simulink model "bicycle_sim11"  (Simulink 8.7)
settings: Solver=VariableStepAuto  SolverMode=SingleTasking  StartTime=0.0  StopTime=30  RelTol=1e-3
values from neighbouring files (symbols this model uses):
  a = 4    [bicycle.m]    (also in diff_drive.m)
  d = 0.01    [bicycle.m]    (also in diff_drive.m = 0.075)
  K_theta = 1    [bicycle.m]    (also in diff_drive.m = 0.001)
  Kp = 7    [bicycle.m]    (also in diff_drive.m = 1)
  Kx = 30    [bicycle.m]    (also in diff_drive.m = 15)
  Ky = 30    [bicycle.m]    (also in diff_drive.m = 150)
  theta0 = pi/2    (= 1.57079632679)    [bicycle.m]    (also in diff_drive.m)
  w = 0.1    [bicycle.m]    (also in diff_drive.m)
  x0 = a    (= 4)    [bicycle.m]    (also in diff_drive.m)
  y0 = 0    [bicycle.m]    (also in diff_drive.m)
libraries: simulink_extras x2
settings Model: Creator=olivier  LastModifiedBy=sanjy
settings SolverCC: ZeroCrossAlgorithm=Adaptive
settings DataIOCC: LimitDataPoints=off  SaveFormat=Dataset
settings DebuggingCC: UnderspecifiedInitializationDetection=Simplified  MergeDetectMultiDrivingBlocksExec=error  MaskedZcDiagnostic=none  SFUnexpectedBacktrackingDiag=error  SFNoUnconditionalDefaultTransitionDiag=error
settings HardwareCC: ProdBitPerPointer=64  ProdLargestAtomicFloat=Float  ProdIntDivRoundTo=Zero  ProdEndianess=LittleEndian  ProdWordSize=64  ProdHWDeviceType=Intel->x86-64 (Windows64)
settings ModelReferenceCC: PropagateSignalLabelsOutOfModel=on
settings SFSimCC: SimUseLocalCustomCode=on
settings RTWCC: RTWUseLocalCustomCode=on
settings GRTTargetCC: TargetLangStandard=C99 (ISO)  GeneratePreprocessorConditionals=Use local settings
settings ConfigComp: CovMetricSettings=dwe  CovHtmlReporting=off  CovSaveCumulativeToWorkspaceVar=off  CovSaveSingleToWorkspaceVar=off  CovModelRefEnable=off  CovExternalEMLEnable=on

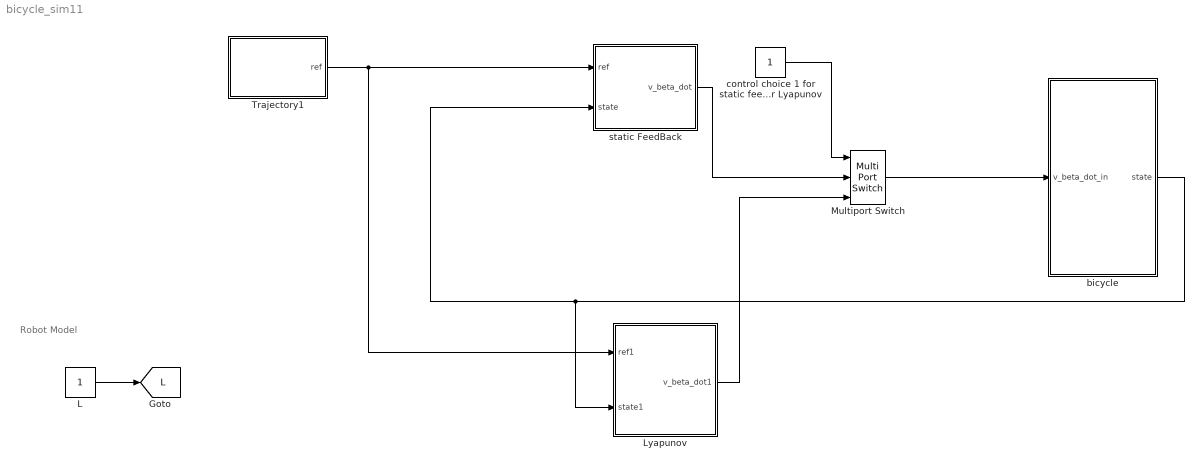
== system bicycle_sim11 ==
  note: Robot Model
  L : Constant
  Lyapunov : Subsystem
  Multiport Switch : MultiPortSwitch  Inputs=2
  Trajectory1 : Subsystem  TreatAsAtomicUnit=on
  bicycle : Subsystem  mask{L_error=0, radius_error=0, omega_max=100, beta_max=45, beta_dot_max=50}
      mask prompts: L_error "L error in percent"; radius_error "Radius error in percent"; omega_max "Max Rotation Velocity"; beta_max "Max Orientation"; beta_dot_max "Max Orientation Velocity"
  control choice 1 for static feedback 2 for Lyapunov : Constant
  static FeedBack : Subsystem
  tag scope: L=global
  wires:
  Lyapunov/1(v_beta_dot1) -> Multiport Switch/3
  L/1 -> [L]
  bicycle/1(state) -> Lyapunov/2(state1), static FeedBack/2(state)
  control choice 1 for static feedback 2 for Lyapunov/1 -> Multiport Switch/1
  Multiport Switch/1 -> bicycle/1(v_beta_dot_in)
  static FeedBack/1(v_beta_dot) -> Multiport Switch/2
  Trajectory1/1(ref) -> Lyapunov/1(ref1), static FeedBack/1(ref)

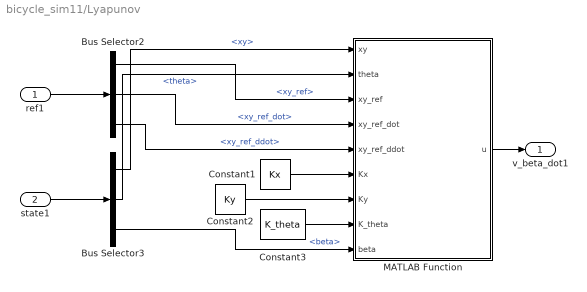
== system bicycle_sim11/Lyapunov ==
  ref1 : Inport
  state1 : Inport  Port=2
  Bus Selector2 : BusSelector  OutputSignals=xy_ref,xy_ref_dot,xy_ref_ddot
  Bus Selector3 : BusSelector  OutputSignals=xy,theta,beta
  Constant1 : Constant  Value=Kx
  Constant2 : Constant  Value=Ky
  Constant3 : Constant  Value=K_theta
  MATLAB Function : MATLAB Function  TreatAsAtomicUnit=on
  v_beta_dot1 : Outport
  wires:
  Constant3/1 -> MATLAB Function/8(K_theta)
  Constant2/1 -> MATLAB Function/7(Ky)
  Constant1/1 -> MATLAB Function/6(Kx)
  Bus Selector3/2 -> MATLAB Function/2(theta)  "<theta>"
  Bus Selector2/1 -> MATLAB Function/3(xy_ref)  "<xy_ref>"
  Bus Selector3/1 -> MATLAB Function/1(xy)  "<xy>"
  Bus Selector2/2 -> MATLAB Function/4(xy_ref_dot)  "<xy_ref_dot>"
  MATLAB Function/1(u) -> v_beta_dot1/1
  state1/1 -> Bus Selector3/1
  Bus Selector2/3 -> MATLAB Function/5(xy_ref_ddot)  "<xy_ref_ddot>"
  ref1/1 -> Bus Selector2/1
  Bus Selector3/3 -> MATLAB Function/9(beta)  "<beta>"

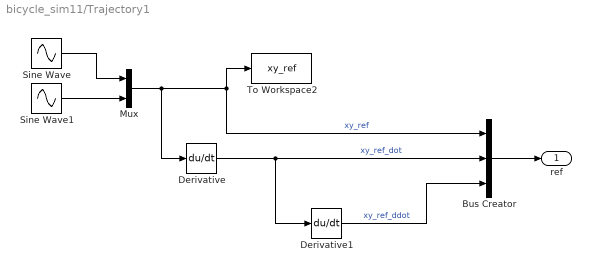
== system bicycle_sim11/Trajectory1 ==
  Bus Creator : BusCreator  Inputs=3
  Derivative : Derivative
  Derivative1 : Derivative
  Mux : Mux  Inputs=2
  Sine Wave : Sin  Amplitude=a  Frequency=w  Phase=pi/2  SampleTime=0
  Sine Wave1 : Sin  Amplitude=a  Frequency=w  SampleTime=0
  To Workspace2 : ToWorkspace  VariableName=xy_ref  SampleTime=-1
      settings: Save2DSignal=2-D array (concatenate along first dimension)
  ref : Outport
  wires:
  Bus Creator/1 -> ref/1
  Mux/1 -> Derivative/1, Bus Creator/1, To Workspace2/1  "xy_ref"
  Derivative/1 -> Bus Creator/2, Derivative1/1  "xy_ref_dot"
  Derivative1/1 -> Bus Creator/3  "xy_ref_ddot"
  Sine Wave1/1 -> Mux/2
  Sine Wave/1 -> Mux/1

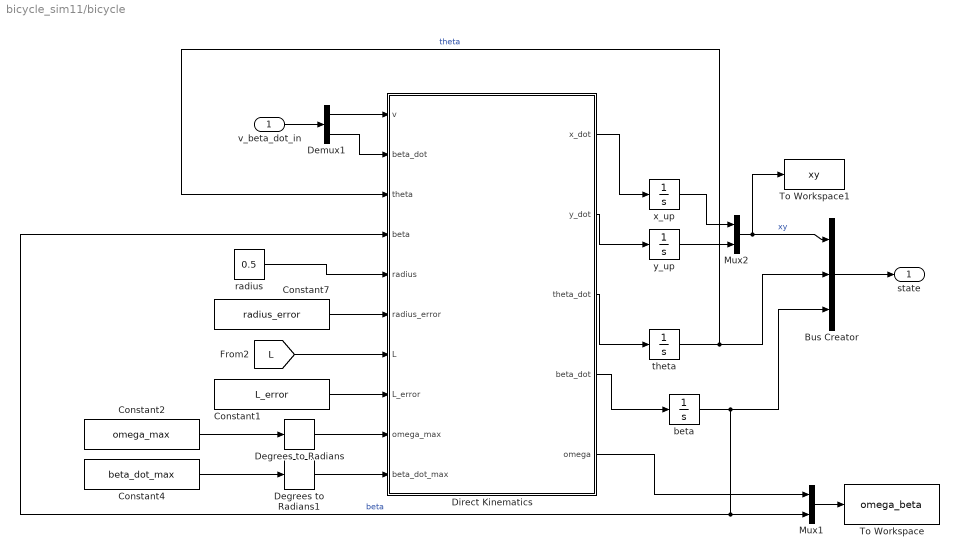
== system bicycle_sim11/bicycle ==
  v_beta_dot_in : Inport
  Bus Creator : BusCreator  Inputs=3
  Constant1 : Constant  Value=L_error
  Constant2 : Constant  Value=omega_max
  Constant4 : Constant  Value=beta_dot_max
  Constant7 : Constant  Value=radius_error
  Degrees to Radians : simulink_extras/Transformations/Degrees to Radians
  Degrees to Radians1 : simulink_extras/Transformations/Degrees to Radians
  Demux1 : Demux  Outputs=2
  Direct Kinematics : MATLAB Function  TreatAsAtomicUnit=on
  Mux1 : Mux  Inputs=2
  Mux2 : Mux  Inputs=2
  To Workspace : ToWorkspace  VariableName=omega_beta  SampleTime=-1
      settings: Save2DSignal=2-D array (concatenate along first dimension)
  To Workspace1 : ToWorkspace  VariableName=xy  SampleTime=-1
      settings: Save2DSignal=2-D array (concatenate along first dimension)
  beta : Integrator  LimitOutput=on  UpperSaturationLimit=beta_max*pi/180  LowerSaturationLimit=-beta_max*pi/180
  radius : Constant  Value=0.5
  theta : Integrator  InitialCondition=theta0
  x_up : Integrator  InitialCondition=x0
  y_up : Integrator  InitialCondition=y0
  state : Outport
  wires:
  Direct Kinematics/2(y_dot) -> y_up/1
  Direct Kinematics/1(x_dot) -> x_up/1
  x_up/1 -> Mux2/1
  y_up/1 -> Mux2/2
  Mux2/1 -> Bus Creator/1, To Workspace1/1  "xy"
  Bus Creator/1 -> state/1
  v_beta_dot_in/1 -> Demux1/1
  Demux1/1 -> Direct Kinematics/1(v)
  [L] -> Direct Kinematics/7(L)
  Constant1/1 -> Direct Kinematics/8(L_error)
  Constant7/1 -> Direct Kinematics/6(radius_error)
  Direct Kinematics/3(theta_dot) -> theta/1
  Direct Kinematics/4(beta_dot) -> beta/1
  theta/1 -> Direct Kinematics/3(theta), Bus Creator/2  "theta"
  beta/1 -> Direct Kinematics/4(beta), Mux1/2, Bus Creator/3  "beta"
  Constant2/1 -> Degrees to Radians/1
  Constant4/1 -> Degrees to Radians1/1
  Direct Kinematics/5(omega) -> Mux1/1
  Mux1/1 -> To Workspace/1
  radius/1 -> Direct Kinematics/5(radius)
  Demux1/2 -> Direct Kinematics/2("beta_dot ")
  Degrees to Radians/1 -> Direct Kinematics/9(omega_max)
  Degrees to Radians1/1 -> Direct Kinematics/10(beta_dot_max)

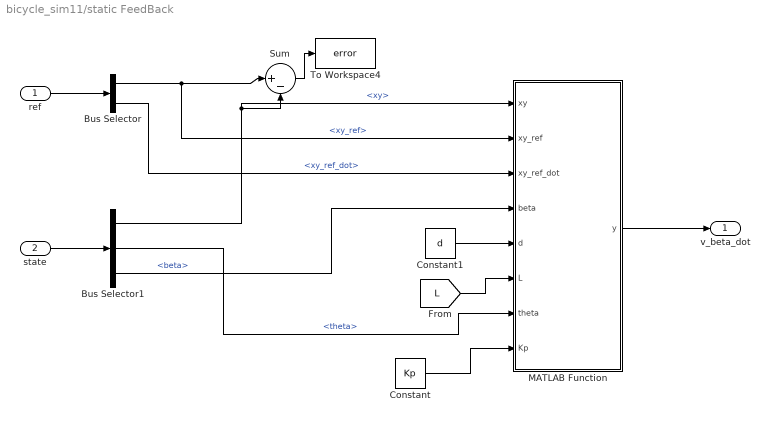
== system bicycle_sim11/static FeedBack ==
  ref : Inport
  state : Inport  Port=2
  Bus Selector : BusSelector  OutputSignals=xy_ref,xy_ref_dot
  Bus Selector1 : BusSelector  OutputSignals=xy,theta,beta
  Constant : Constant  Value=Kp
  Constant1 : Constant  Value=d
  MATLAB Function : MATLAB Function  TreatAsAtomicUnit=on
  Sum : Sum  Inputs=|+-
  To Workspace4 : ToWorkspace  VariableName=error  SampleTime=-1
      settings: Save2DSignal=2-D array (concatenate along first dimension)
  v_beta_dot : Outport
  wires:
  Sum/1 -> To Workspace4/1
  ref/1 -> Bus Selector/1
  state/1 -> Bus Selector1/1
  Bus Selector/1 -> MATLAB Function/2(xy_ref), Sum/1  "<xy_ref>"
  Bus Selector1/1 -> MATLAB Function/1(xy), Sum/2  "<xy>"
  Constant1/1 -> MATLAB Function/5(d)
  [L] -> MATLAB Function/6(L)
  Bus Selector/2 -> MATLAB Function/3(xy_ref_dot)  "<xy_ref_dot>"
  Bus Selector1/3 -> MATLAB Function/4(beta)  "<beta>"
  Bus Selector1/2 -> MATLAB Function/7(theta)  "<theta>"
  Constant/1 -> MATLAB Function/8(Kp)
  MATLAB Function/1(y) -> v_beta_dot/1

== matlab function bicycle/Direct Kinematics ==
  data: v input double; beta_dot input double; x_dot output double; theta input double; beta input double; radius input double; radius_error input double; L input double; L_error input double; omega_max input double; beta_dot_max input double; y_dot output double; theta_dot output double; beta_dot output double; omega output double
function [x_dot, y_dot, theta_dot, beta_dot, omega]  = dk(v, beta_dot, theta, beta, radius, radius_error, L, L_error, omega_max, beta_dot_max)

% commanded wheel rotation velocity
omega = v/radius;
omega = max(-omega_max, min(omega, omega_max));

% actual linear velocity
v = (1+radius_error*0.01)*radius * omega;

% actual L value
L = (1+L_error*0.01)*L;

x_dot = v*cos(theta)*cos(beta);
y_dot = v*sin(theta)*cos(beta);
theta_dot = v*sin(beta)/L;
beta_dot = max(-beta_dot_max, min(beta_dot, beta_dot_max));

== matlab function static FeedBack/MATLAB Function ==
  data: xy input double; y output double; xy_ref input double; xy_ref_dot input double; beta input double; d input double; L input double; theta input double; Kp input double
function y = fcn(xy,xy_ref,xy_ref_dot,beta,d,L,theta,Kp)
%#codegen
%% calculate Xp
xp = xy(1) + L * cos(theta) +d * cos(theta+beta);
yp= xy(end) + L * sin(theta) + d * sin(theta + beta);

Xp= [xp;yp];

%% Error 
error = xy_ref - Xp;

%% Calculate K mayrix and inverse
K= [cos(theta + beta) - (d/L)*sin(beta)*sin(theta + beta), -d*sin(theta + beta) ;
     sin(theta + beta) + (d/L)*sin(beta)*cos(theta + beta),  d*cos(theta + beta) ] ;
 
K_inv= inv(K);
%%  find controlled inputs

y = K_inv * (xy_ref_dot + Kp*error); 
%%

== matlab function Lyapunov/MATLAB Function ==
  data: xy input double; u output double; theta input double; xy_ref input double; xy_ref_dot input double; xy_ref_ddot input double; Kx input double; Ky input double; K_theta input double; beta input double
function u = fcn(xy,theta,xy_ref,xy_ref_dot,xy_ref_ddot,Kx,Ky,K_theta,beta)

xe = cos(theta)*(xy_ref(1)-xy(1)-(L*cos(theta))) + sin(theta)*(xy_ref(2)-xy(end)-(L*sin(theta)));

ye = -sin(theta)*(xy_ref(1)-xy(1)-(L*cos(theta))) + cos(theta)*(xy_ref(2)-xy(end)-(L*sin(theta)));

theta_e = atan2(xy_ref_dot(2),xy_ref_dot(1)) - theta - beta;

theta_e = theta_e -2*pi*floor((theta_e+pi)/(2*pi));

vr = (xy_ref_dot(1)*cos(theta)) + (xy_ref_dot(2)*sin(theta));

if vr == 0
    
    wr = 0;
    
else
    
wr = (xy_ref_dot(1)*xy_ref_ddot(2) - xy_ref_ddot(1)*xy_ref_dot(2))/vr^2;

end

v = vr*cos(theta_e) + Kx*xe;

w = wr + (Ky*ye*vr*sin(theta_e)/theta_e) + (K_theta*theta_e);

beta_dot = w - ((v*sin(beta))/L);

u = [v;beta_dot];
